simulink model "SingleAgent_Pendulum"  (R2018b)
settings: Solver=VariableStepAuto  StartTime=0.0  StopTime=10  RelTol=1e-3
undefined symbols (not defined in the file or in its folder): p02, q01
settings Model: Creator=oscar  LastModifiedBy=oscar
settings DataIOCC: OutputOption=SpecifiedOutputTimes  OutputTimes=t_out

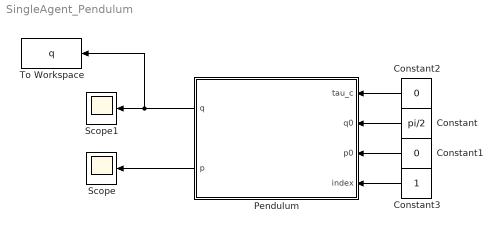
== system SingleAgent_Pendulum ==
  Constant : Constant  Value=pi/2
  Constant1 : Constant  Value=0
  Constant2 : Constant  Value=0
  Constant3 : Constant
  Pendulum : Subsystem
  Scope : Scope
  Scope1 : Scope
  To Workspace : ToWorkspace  VariableName=q  SaveFormat=Timeseries  SampleTime=-1
  wires:
  Constant/1 -> Pendulum/2(q0)
  Constant1/1 -> Pendulum/3(p0)
  Pendulum/2(p) -> Scope/1
  Pendulum/1(q) -> To Workspace/1, Scope1/1
  Constant3/1 -> Pendulum/4(index)
  Constant2/1 -> Pendulum/1(tau_c)

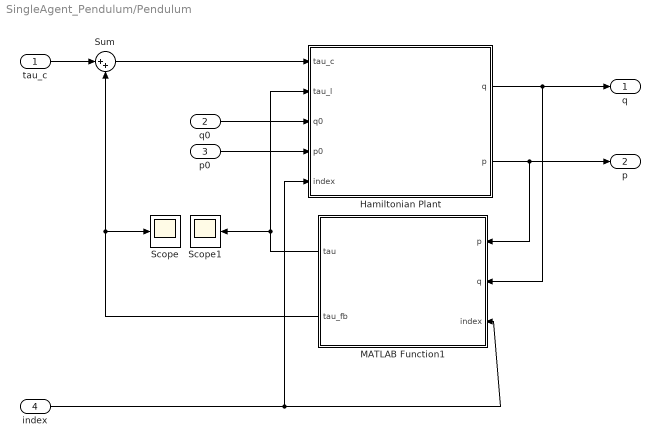
== system SingleAgent_Pendulum/Pendulum ==
  tau_c : Inport
  q0 : Inport  Port=2
  p0 : Inport  Port=3
  index : Inport  Port=4
  Hamiltonian Plant : Subsystem
  MATLAB Function1 : MATLAB Function  TreatAsAtomicUnit=on
  Scope : Scope
  Scope1 : Scope
  Sum : Sum  Inputs=|++
  q : Outport
  p : Outport  Port=2
  wires:
  MATLAB Function1/1(tau) -> Scope1/1, Hamiltonian Plant/2(tau_l)
  tau_c/1 -> Sum/1
  Hamiltonian Plant/2(p) -> p/1, MATLAB Function1/1(p)
  Hamiltonian Plant/1(q) -> MATLAB Function1/2(q), q/1
  q0/1 -> Hamiltonian Plant/3(q0)
  p0/1 -> Hamiltonian Plant/4(p0)
  MATLAB Function1/2(tau_fb) -> Scope/1, Sum/2
  Sum/1 -> Hamiltonian Plant/1(tau_c)
  index/1 -> Hamiltonian Plant/5(index), MATLAB Function1/3(index)

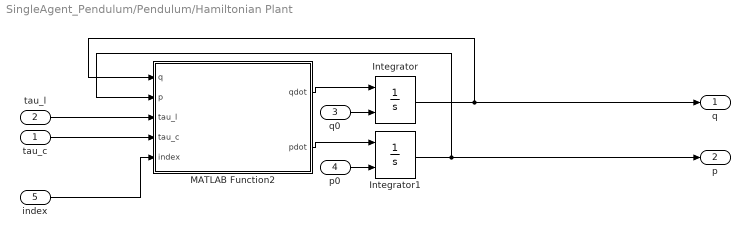
== system SingleAgent_Pendulum/Pendulum/Hamiltonian Plant ==
  tau_c : Inport
  tau_l : Inport  Port=2
  q0 : Inport  Port=3
  p0 : Inport  Port=4
  index : Inport  Port=5
  Integrator : Integrator  InitialConditionSource=external  InitialCondition=q01
  Integrator1 : Integrator  InitialConditionSource=external  InitialCondition=p02
  MATLAB Function2 : MATLAB Function  TreatAsAtomicUnit=on
  q : Outport
  p : Outport  Port=2
  wires:
  tau_l/1 -> MATLAB Function2/3(tau_l)
  MATLAB Function2/2(pdot) -> Integrator1/1
  Integrator1/1 -> MATLAB Function2/2(p), p/1
  Integrator/1 -> MATLAB Function2/1(q), q/1
  MATLAB Function2/1(qdot) -> Integrator/1
  p0/1 -> Integrator1/2
  tau_c/1 -> MATLAB Function2/4(tau_c)
  q0/1 -> Integrator/2
  index/1 -> MATLAB Function2/5(index)

== matlab function SingleAgent_Pendulum/Pendulum/Hamiltonian Plant/MATLAB Function2 ==
  data: q input; qdot output; p input; tau_l input; pdot output; tau_c input; index input
function [qdot, pdot] = fcn(q, p, tau_l, tau_c, index)

    coder.extrinsic('Pendulum_Dynamics');
    qdot = 0;
    pdot = 0;
    [qdot, pdot] = Pendulum_Dynamics(q, p, tau_l, tau_c, index);

== matlab function SingleAgent_Pendulum/Pendulum/MATLAB Function1 ==
  data: p input; q input; tau output; tau_fb output; index input
function [tau, tau_fb] = LocalControl(p, q, index)
    

coder.extrinsic('Pendulum_Control');
tau = 0;
tau_fb = 0;
[tau, tau_fb] = Pendulum_Control(q, p, index);
